simulink model "PMSM_Plant_Model"  (R2020a)
settings: configuration reference "SLRT" (kept outside this file)
undefined symbols (not defined in the file): adcTransducerVoltAtZeroAmpere, adcTransducerVoltPerAmpere, discInertia, encoderCountPerRevolution, encoderPositionValidAtStartup, encoderRotorPositionAtIndex, inverterBusVoltage, pmsmCoulombFrictionTorque, pmsmInductanceL0, pmsmInertia, pmsmPolePairs, pmsmRotorPositionInit, pmsmTorqueConstant, pmsmViscousFrictionCoefficient, pwmCounterMax, sampleTimeCurrentControl
libraries: fl_lib x15, nesl_utility x14, ee_lib x6, autolibpmsmexterior x2, utils_lib x1, mcbplantlib x1, autolibinverter x1, RotationalFrictionBrake_lib x1, eeTransforms x1
settings Model: DataDictionary=pmsmPlantData.sldd  EnableAccessToBaseWorkspace=off  DataTypeOverride=Off  VariantConfigurationObject=pmsmPlantVarObj  OrderedModelArguments=off  Creator=promero  LastModifiedBy=manuel.fedou
settings ConfigSetRef: SourceName=SLRT

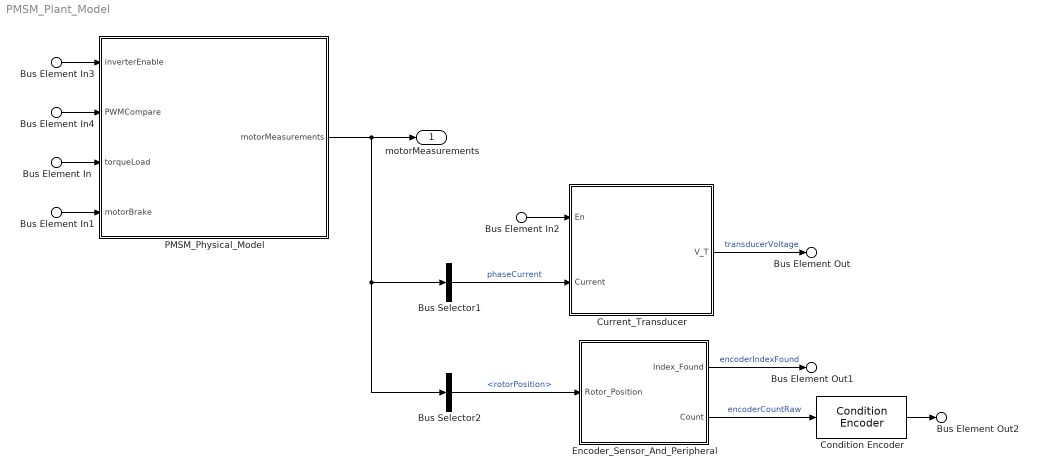
== system PMSM_Plant_Model ==
  Bus Element In : Inport  PortName=inputs  Element=torqueLoad
  Bus Element In2 : Inport  PortName=inputs  Element=connectCurrentSensor
  Bus Element In1 : Inport  PortName=inputs  Element=motorBrake
  Bus Element In3 : Inport  Port=2  PortName=commands  Element=inverterEnable
  Bus Element In4 : Inport  Port=2  PortName=commands  Element=pwmCompare
  Bus Selector1 : BusSelector  OutputSignals=phaseCurrentA,phaseCurrentB  OutputAsBus=on
  Bus Selector2 : BusSelector  OutputSignals=rotorPosition
  Condition Encoder : utils_lib/Condition Encoder  cntsPerRevolution=encoderCountPerRevolution  positiveDirection=encoderALeadsB
  Current_Transducer : Subsystem
      mask Display: image('currentTransducerMask.png');
  Encoder_Sensor_And_Peripheral : Subsystem
      mask Display:
      | image('encoderSensorAndPeripheralMask.png')
      | port_label('input',1,'P')
      | port_label('output',1,sprintf('Index\nFound'))
      | port_label('output',2,'Count')
  PMSM_Physical_Model : Subsystem  Variant=on  VariantControl=Choice
      mask Display: image('focVelocityMotorAndLoadMask.png'); % Use "Edit Image" on toolstrip to change.
  motorMeasurements : Outport  OutDataTypeStr=Bus: motorMeasurements  VectorParamsAs1DForOutWhenUnconnected=off
  Bus Element Out : Outport  Port=2  PortName=feedback  Element=transducerVoltage
  Bus Element Out1 : Outport  Port=2  PortName=feedback  Element=encoderIndexFound
  Bus Element Out2 : Outport  Port=2  PortName=feedback  Element=encoderCount
  wires:
  Bus Selector2/1 -> Encoder_Sensor_And_Peripheral/1(Rotor_Position)  "<rotorPosition>"
  Encoder_Sensor_And_Peripheral/2(Count) -> Condition Encoder/1  "encoderCountRaw"
  PMSM_Physical_Model/1(motorMeasurements) -> motorMeasurements/1, Bus Selector2/1, Bus Selector1/1
  Bus Element In3/1 -> PMSM_Physical_Model/1(inverterEnable)
  Bus Element In4/1 -> PMSM_Physical_Model/2(PWMCompare)
  Bus Selector1/1 -> Current_Transducer/2(Current)  "phaseCurrent"
  Bus Element In/1 -> PMSM_Physical_Model/3(torqueLoad)
  Bus Element In1/1 -> PMSM_Physical_Model/4(motorBrake)
  Bus Element In2/1 -> Current_Transducer/1(En)
  Current_Transducer/1(V_T) -> Bus Element Out/1  "transducerVoltage"
  Encoder_Sensor_And_Peripheral/1(Index_Found) -> Bus Element Out1/1  "encoderIndexFound"
  Condition Encoder/1 -> Bus Element Out2/1

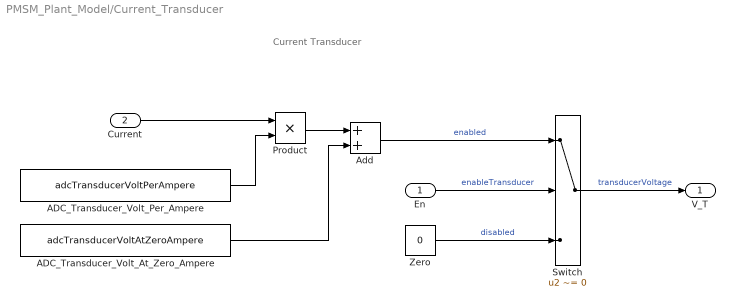
== system PMSM_Plant_Model/Current_Transducer ==
  note: Current Transducer
  En : Inport
  Current : Inport  Port=2
  ADC_Transducer_Volt_At_Zero_Ampere : Constant  Value=adcTransducerVoltAtZeroAmpere
  ADC_Transducer_Volt_Per_Ampere : Constant  Value=adcTransducerVoltPerAmpere
  Add : Sum
  Product : Product  RndMeth=Zero
  Switch : Switch  Criteria=u2 ~= 0  OutDataTypeStr=Inherit: Inherit via back propagation
  Zero : Constant  Value=0
  V_T : Outport  VectorParamsAs1DForOutWhenUnconnected=off
  wires:
  Current/1 -> Product/1
  ADC_Transducer_Volt_At_Zero_Ampere/1 -> Add/2
  Product/1 -> Add/1
  ADC_Transducer_Volt_Per_Ampere/1 -> Product/2
  Zero/1 -> Switch/3  "disabled"
  Switch/1 -> V_T/1  "transducerVoltage"
  Add/1 -> Switch/1  "enabled"
  En/1 -> Switch/2  "enableTransducer"

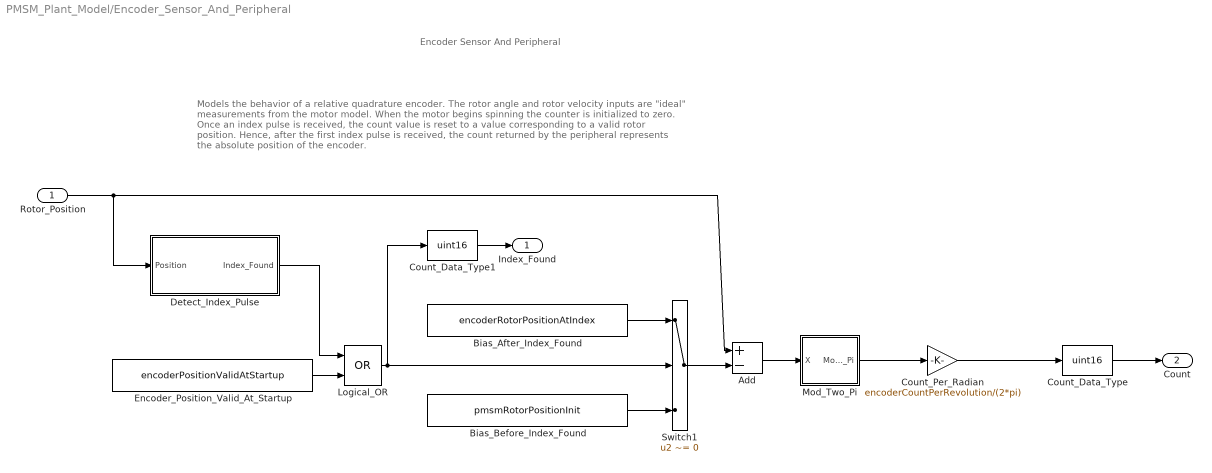
== system PMSM_Plant_Model/Encoder_Sensor_And_Peripheral ==
  note: Models the behavior of a relative quadrature encoder. The rotor angle and rotor velocity inputs are "ideal" measurements from the motor model.
      | When the motor begins spinning the counter is initialized to zero.
      | Once an index pulse is received, the count value is reset to a value corresponding to a valid rotor position.
      | Hence, after the first index pulse is received, the count returned by the peripheral represents the absolute position of the encoder.
  note: Encoder Sensor And Peripheral
  Rotor_Position : Inport
  Add : Sum  Inputs=+-
  Bias_After_Index_Found : Constant  Value=encoderRotorPositionAtIndex
  Bias_Before_Index_Found : Constant  Value=pmsmRotorPositionInit
  Count_Data_Type : DataTypeConversion  OutDataTypeStr=uint16
  Count_Data_Type1 : DataTypeConversion  OutDataTypeStr=uint16
  Count_Per_Radian : Gain  Gain=encoderCountPerRevolution/(2*pi)
      settings: AttributesFormatString=|
      | ------------------------------------------
      | Gain = %<Gain>
  Detect_Index_Pulse : Subsystem
  Encoder_Position_Valid_At_Startup : Constant  Value=encoderPositionValidAtStartup
  Logical_OR : Logic  Operator=OR  IconShape=distinctive  AllPortsSameDT=off  OutDataTypeStr=boolean
  Mod_Two_Pi : Subsystem
      mask Display:
      | text(0.5, 0.5,'Mod 2\pi',...
      |   'HorizontalAlignment', 'Center',...
      |   'VerticalAlignment', 'Middle',...
      |   'texmode', 'on')
  Switch1 : Switch  Criteria=u2 ~= 0
  Index_Found : Outport  VectorParamsAs1DForOutWhenUnconnected=off
  Count : Outport  Port=2  VectorParamsAs1DForOutWhenUnconnected=off
  wires:
  Bias_Before_Index_Found/1 -> Switch1/3
  Bias_After_Index_Found/1 -> Switch1/1
  Logical_OR/1 -> Count_Data_Type1/1, Switch1/2
  Encoder_Position_Valid_At_Startup/1 -> Logical_OR/2
  Detect_Index_Pulse/1(Index_Found) -> Logical_OR/1
  Rotor_Position/1 -> Add/1, Detect_Index_Pulse/1(Position)
  Mod_Two_Pi/1(Mod_X_Two_Pi) -> Count_Per_Radian/1
  Count_Data_Type/1 -> Count/1
  Switch1/1 -> Add/2
  Add/1 -> Mod_Two_Pi/1(X)
  Count_Per_Radian/1 -> Count_Data_Type/1
  Count_Data_Type1/1 -> Index_Found/1

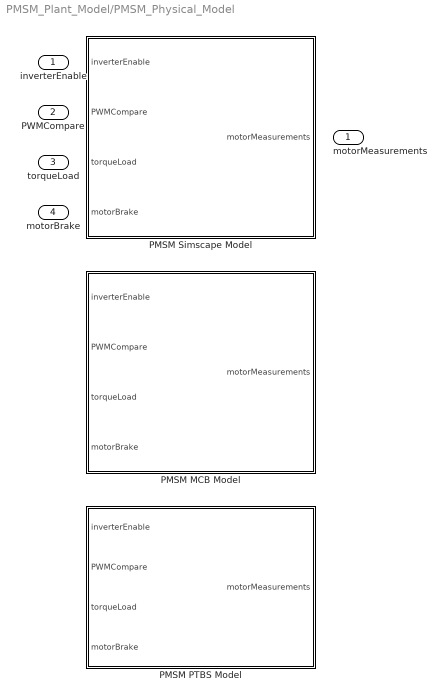
== system PMSM_Plant_Model/PMSM_Physical_Model ==
  inverterEnable : Inport
  PWMCompare : Inport  Port=2
  torqueLoad : Inport  Port=3
  motorBrake : Inport  Port=4
  PMSM MCB Model : Subsystem  VariantControl=MCBPlant
  PMSM PTBS Model : Subsystem  VariantControl=PTBSPlant
  PMSM Simscape Model : Subsystem  VariantControl=SimscapePlant
  motorMeasurements : Outport

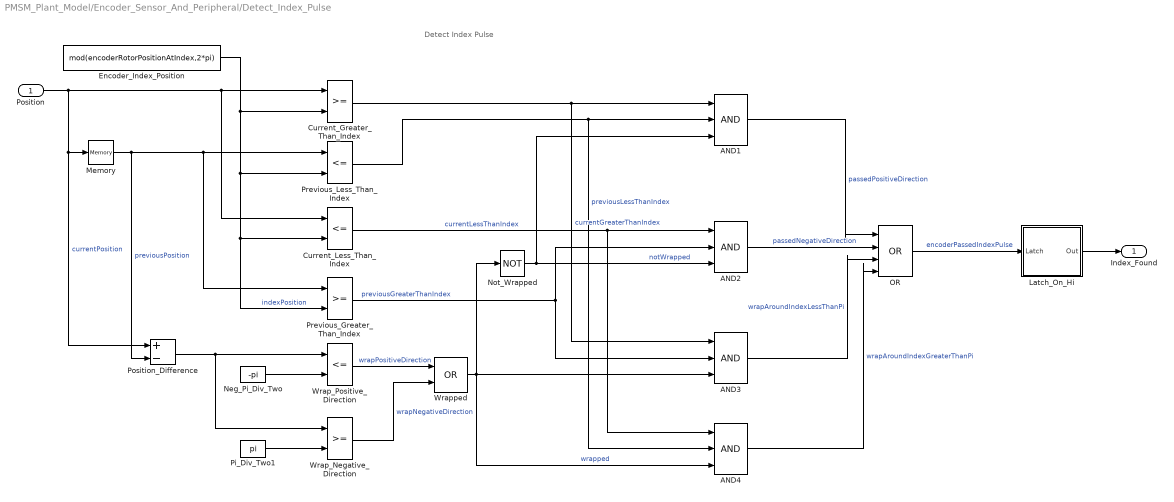
== system PMSM_Plant_Model/Encoder_Sensor_And_Peripheral/Detect_Index_Pulse ==
  note: Detect Index Pulse
  Position : Inport
  AND{1..4} (4 alike) : Logic  Inputs=3  IconShape=distinctive  AllPortsSameDT=off  OutDataTypeStr=boolean
  Current_Greater_Than_Index : RelationalOperator  OutDataTypeStr=boolean  RndMeth=Nearest
  Current_Less_Than_Index : RelationalOperator  Operator=<=  OutDataTypeStr=boolean  RndMeth=Nearest
  Encoder_Index_Position : Constant  Value=mod(encoderRotorPositionAtIndex,2*pi)
  Latch_On_Hi : Subsystem
  Memory : Memory  InitialCondition=pmsmRotorPositionInit  LinearizeAsDelay=on
  Neg_Pi_Div_Two : Constant  Value=-pi
  Not_Wrapped : Logic  Operator=NOT  IconShape=distinctive  AllPortsSameDT=off  OutDataTypeStr=boolean
  OR : Logic  Operator=OR  Inputs=4  IconShape=distinctive  AllPortsSameDT=off  OutDataTypeStr=boolean
  Pi_Div_Two1 : Constant  Value=pi
  Position_Difference : Sum  Inputs=+-
  Previous_Greater_Than_Index : RelationalOperator  OutDataTypeStr=boolean  RndMeth=Nearest
  Previous_Less_Than_Index : RelationalOperator  Operator=<=  OutDataTypeStr=boolean  RndMeth=Nearest
  Wrap_Negative_Direction : RelationalOperator  OutDataTypeStr=boolean  RndMeth=Nearest
  Wrap_Positive_Direction : RelationalOperator  Operator=<=  OutDataTypeStr=boolean  RndMeth=Nearest
  Wrapped : Logic  Operator=OR  IconShape=distinctive  AllPortsSameDT=off  OutDataTypeStr=boolean
  Index_Found : Outport  VectorParamsAs1DForOutWhenUnconnected=off
  wires:
  AND2/1 -> OR/2  "passedNegativeDirection"
  AND1/1 -> OR/1  "passedPositiveDirection"
  Current_Less_Than_Index/1 -> AND2/1, AND4/1  "currentLessThanIndex"
  Previous_Greater_Than_Index/1 -> AND2/2, AND3/2  "previousGreaterThanIndex"
  OR/1 -> Latch_On_Hi/1(Latch)  "encoderPassedIndexPulse"
  Encoder_Index_Position/1 -> Previous_Less_Than_Index/2, Previous_Greater_Than_Index/2, Current_Less_Than_Index/2, Current_Greater_Than_Index/2  "indexPosition"
  Previous_Less_Than_Index/1 -> AND1/2, AND4/2  "previousLessThanIndex"
  Current_Greater_Than_Index/1 -> AND3/1, AND1/1  "currentGreaterThanIndex"
  Memory/1 -> Position_Difference/2, Previous_Greater_Than_Index/1, Previous_Less_Than_Index/1  "previousPosition"
  Position/1 -> Memory/1, Position_Difference/1, Current_Less_Than_Index/1, Current_Greater_Than_Index/1  "currentPosition"
  Position_Difference/1 -> Wrap_Negative_Direction/1, Wrap_Positive_Direction/1
  Wrap_Positive_Direction/1 -> Wrapped/1  "wrapPositiveDirection"
  Neg_Pi_Div_Two/1 -> Wrap_Positive_Direction/2
  Wrap_Negative_Direction/1 -> Wrapped/2  "wrapNegativeDirection"
  Pi_Div_Two1/1 -> Wrap_Negative_Direction/2
  AND3/1 -> OR/3  "wrapAroundIndexLessThanPi"
  Latch_On_Hi/1(Out) -> Index_Found/1
  Not_Wrapped/1 -> AND1/3, AND2/3  "notWrapped"
  Wrapped/1 -> AND4/3, AND3/3, Not_Wrapped/1  "wrapped"
  AND4/1 -> OR/4  "wrapAroundIndexGreaterThanPi"

== system PMSM_Plant_Model/Encoder_Sensor_And_Peripheral/Mod_Two_Pi ==
  note: Mod Two Pi
  X : Inport
  Mod : Math  Operator=mod  SignedPower=on  SaturateOnIntegerOverflow=on
  Two_Pi : Constant  Value=2*pi  OutDataTypeStr=Inherit: Inherit via back propagation
  Mod_X_Two_Pi : Outport  VectorParamsAs1DForOutWhenUnconnected=off
  wires:
  X/1 -> Mod/1
  Two_Pi/1 -> Mod/2
  Mod/1 -> Mod_X_Two_Pi/1

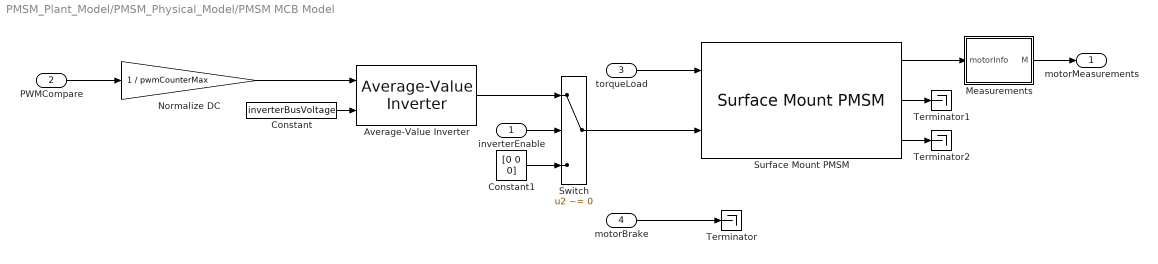
== system PMSM_Plant_Model/PMSM_Physical_Model/PMSM MCB Model ==
  inverterEnable : Inport
  PWMCompare : Inport  Port=2
  torqueLoad : Inport  Port=3
  motorBrake : Inport  Port=4
  Average-Value Inverter : mcbplantlib/Average-Value Inverter
  Constant : Constant  Value=inverterBusVoltage
  Constant1 : Constant  Value=[0 0 0]
  Measurements : Subsystem
  Normalize DC : Gain  Gain=1 / pwmCounterMax  OutDataTypeStr=double
  Surface Mount PMSM : autolibpmsmexterior/Surface Mount PMSM  port_config=Torque  sim_type=Discrete  Ts=sampleTimeCurrentControl  P=pmsmPolePairs  Rs=pmsmStatorPhaseResistance  Ldq_=pmsmInductanceLd  KConstText=Torque constant (Kt):  lambda_pm=pmsmFluxLinkage  Ke=159.9771  Kt=pmsmTorqueConstant  mechanical=[pmsmInertia+discInertia, pmsmViscousFrictionCoefficient, pmsmCoulombFrictionTorque]  idq0=[pmsmInductanceL0 pmsmInductanceL0]  theta_init=pmsmRotorPositionInit - 2*pi  omega_init=pmsmRotorVelocityInit  KConst=pmsmTorqueConstant  lambda_pm_calc=0.005  RefBlkName='autolibpmsmexterior/Surface Mount PMSM'  aMode=5  Ldq="[0.0017      0.0017]"
      settings: SourceProductBaseCode=PW,MT,UV,VE,VP
  Switch : Switch  Criteria=u2 ~= 0
  Terminator : Terminator
  Terminator1 : Terminator
  Terminator2 : Terminator
  motorMeasurements : Outport  VectorParamsAs1DForOutWhenUnconnected=off
  wires:
  motorBrake/1 -> Terminator/1
  Surface Mount PMSM/1 -> Measurements/1(motorInfo)
  Measurements/1(M) -> motorMeasurements/1
  inverterEnable/1 -> Switch/2
  Constant1/1 -> Switch/3
  torqueLoad/1 -> Surface Mount PMSM/1
  Constant/1 -> Average-Value Inverter/2
  Switch/1 -> Surface Mount PMSM/2
  Average-Value Inverter/1 -> Switch/1
  Surface Mount PMSM/2 -> Terminator1/1
  Surface Mount PMSM/3 -> Terminator2/1
  Normalize DC/1 -> Average-Value Inverter/1
  PWMCompare/1 -> Normalize DC/1

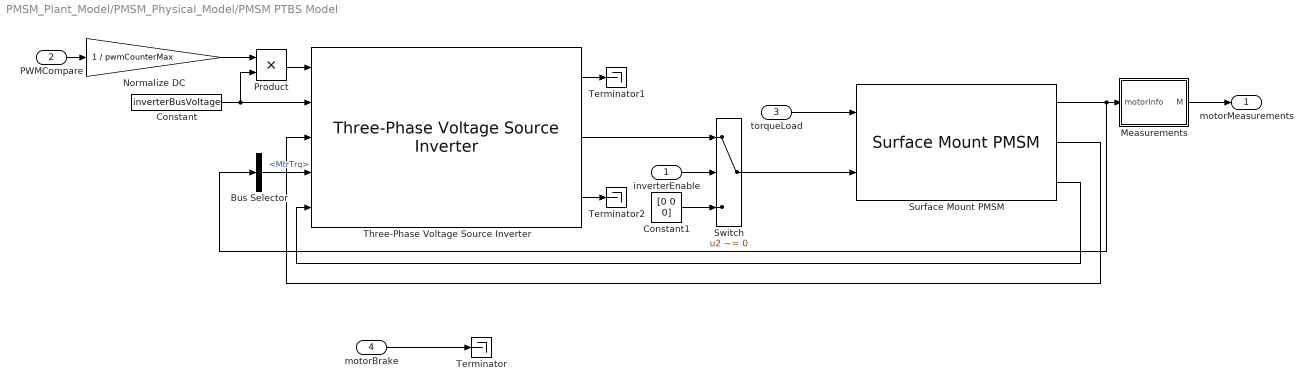
== system PMSM_Plant_Model/PMSM_Physical_Model/PMSM PTBS Model ==
  inverterEnable : Inport
  PWMCompare : Inport  Port=2
  torqueLoad : Inport  Port=3
  motorBrake : Inport  Port=4
  Bus Selector : BusSelector  OutputSignals=MtrTrq
  Constant : Constant  Value=inverterBusVoltage
  Constant1 : Constant  Value=[0 0 0]
  Measurements : Subsystem
  Normalize DC : Gain  Gain=1 / pwmCounterMax  OutDataTypeStr=double
  Product : Product
  Surface Mount PMSM : autolibpmsmexterior/Surface Mount PMSM  port_config=Torque  sim_type=Discrete  Ts=sampleTimeCurrentControl  P=pmsmPolePairs  Rs=pmsmStatorPhaseResistance  Ldq_=pmsmInductanceLd  KConstText=Torque constant (Kt):  lambda_pm=pmsmFluxLinkage  Ke=159.9771  Kt=pmsmTorqueConstant  mechanical=[pmsmInertia+discInertia, pmsmViscousFrictionCoefficient, pmsmCoulombFrictionTorque]  idq0=[pmsmInductanceL0 pmsmInductanceL0]  theta_init=pmsmRotorPositionInit - 2*pi  omega_init=pmsmRotorVelocityInit  KConst=pmsmTorqueConstant  lambda_pm_calc=0.005  RefBlkName='autolibpmsmexterior/Surface Mount PMSM'  aMode=5  Ldq="[0.0017      0.0017]"
      settings: SourceProductBaseCode=PW,MT,UV,VE,VP
  Switch : Switch  Criteria=u2 ~= 0
  Terminator : Terminator
  Terminator1 : Terminator
  Terminator2 : Terminator
  Three-Phase Voltage Source Inverter : autolibinverter/Three-Phase Voltage Source Inverter  InvrtrTmpInpEnbl=off  enable_hdl=off  model_type=Commanded phase voltage  fs=10000  w_eff_bp=[-1000 -500 0 500 1000]  n1=128  T_eff_bp=[-200 -100 0 100 200]  Temp_eff_bp=[213.15 293.15 373.15]  n2=128  ploss_table=[1 0.999 0.989 0.997 0.996;0.995 0.994 0.993 0.992 0.991;0.990 0.989 0.988 0.987 0.986;0.985 0.984 0.983 0.982 0.981;0.980 0.979 0.978 0.977 0.976]  ploss_table_3d=cat(3,0.95*[1 0.999 0.989 0.997 0.996;0.995 0.994 0.993 0.992 0.991;0.990 0.989 0.988 0.987 0.986;0.985 0.984 0.983 0.982 0.981;0.980 0.979 0.978 0.977 0.976],[1 0.999 0.989 0.997 0.996;0.995 0.994 0.993 0.992 0.991;0.990 0.989 0.988 0.987 0.986;0.985 0.984 0.983 0.982 0.981;0.980 0.979 0.978 0.977 0.976],0.92*[1 0.999 0.989 0.997 0.996;0.995 0.994 0.993 0.992 0.991;0.990 0.989 0.988 0.987 0.986;0.985 0.984 0.983 0.982 0.981;0.980 0.979 0.978 0.977 0.976])  preExtrapFlag=off  u1max=1000  u1min=-1000  u2max=200  u2min=-200  intPrec=23  RefBlkName='autolibmappedmotor/Mapped Motor'  CalLossMapData={}  CalLossWithTempMapData={}
      settings: SourceProductBaseCode=PW,MT,UV,VE,VP
  motorMeasurements : Outport  VectorParamsAs1DForOutWhenUnconnected=off
  wires:
  Surface Mount PMSM/2 -> Three-Phase Voltage Source Inverter/3
  inverterEnable/1 -> Switch/2
  Constant1/1 -> Switch/3
  motorBrake/1 -> Terminator/1
  torqueLoad/1 -> Surface Mount PMSM/1
  Switch/1 -> Surface Mount PMSM/2
  PWMCompare/1 -> Normalize DC/1
  Measurements/1(M) -> motorMeasurements/1
  Three-Phase Voltage Source Inverter/2 -> Switch/1
  Surface Mount PMSM/3 -> Three-Phase Voltage Source Inverter/5
  Three-Phase Voltage Source Inverter/1 -> Terminator1/1
  Three-Phase Voltage Source Inverter/3 -> Terminator2/1
  Constant/1 -> Product/2, Three-Phase Voltage Source Inverter/2
  Surface Mount PMSM/1 -> Bus Selector/1, Measurements/1(motorInfo)
  Bus Selector/1 -> Three-Phase Voltage Source Inverter/4  "<MtrTrq>"
  Product/1 -> Three-Phase Voltage Source Inverter/1
  Normalize DC/1 -> Product/1

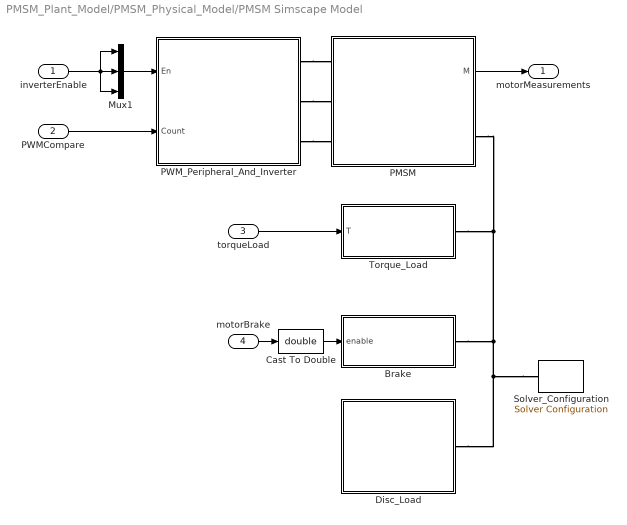
== system PMSM_Plant_Model/PMSM_Physical_Model/PMSM Simscape Model ==
  inverterEnable : Inport
  PWMCompare : Inport  Port=2
  torqueLoad : Inport  Port=3
  motorBrake : Inport  Port=4
  Brake : Subsystem
  Cast To Double : DataTypeConversion  OutDataTypeStr=double
  Disc_Load : Subsystem  VariantControl=loadType == motorLoad.disc
      mask Display: image('discAluminumMask.png')
  Mux1 : Mux  Inputs=3
  PMSM : Subsystem
      mask Display:
      | image('pmsmMask.png')
      | text(0.03, 0.80, 'A', 'HorizontalAlignment', 'Left')
      | text(0.03, 0.50, 'B', 'HorizontalAlignment', 'Left')
      | text(0.03, 0.20, 'C', 'HorizontalAlignment', 'Left')
      | text(0.98, 0.75, 'M', 'HorizontalAlignment', 'Right')
      | text(0.98, 0.25, 'R', 'HorizontalAlignment', 'Right')
  PWM_Peripheral_And_Inverter : Subsystem  VariantControl=variantPwm == enumPwm.behavior
      mask Display: image('pwmPeripheralAndInverterMask.png');
  Solver_Configuration : nesl_utility/Solver Configuration  PhysicalDomain=network_engine_domain  SubClassName=solver  LeftPortType=input  RightPortType=generic  Tones=[]  Harmonics=[]  SimulateNoise=off  Profile=off  UseLocalSampling=off  EnableSwitchedLinearOptims=on  FrequencyDomain=off  UseCCode=off  RelTol=0.001  AbsTol=1e-06  MinStep=1e-09  ToWorkspace=off  RevertToSquareIcSolve=off  NumHomotopyIterations=100  PhasorMode=off  PhasorModeNumHarmonics=1  DoDC=off  ResidualTolerance=1e-9  UseLocalSolver=on  LocalSolverChoice=NE_TRAPEZOIDAL_ADVANCER  LocalSolverSampleTime=sampleTimeCurrentControl  DoFixedCost=on  MaxNonlinIter=1  MaxModeIter=2  LinearAlgebra=auto  EquationFormulation=NE_TIME_EF  DelaysMemoryBudget=1024  AutomaticFiltering=on  FilteringTimeConstant=0.001  PartitionStorageMethod=AS_NEEDED  PartitionMemoryBudget=1024  PartitionMethod=FAST
  Torque_Load : Subsystem  VariantControl=loadType == motorLoad.disc
      mask Display:
      | image('torqueLoadMask.png')
      | text(0.03, 0.5, 'T', 'HorizontalAlignment', 'Left')
      | text(0.98, 0.5, 'R', 'HorizontalAlignment', 'Right')
  motorMeasurements : Outport  VectorParamsAs1DForOutWhenUnconnected=off
  wires:
  PWMCompare/1 -> PWM_Peripheral_And_Inverter/2(Count)
  torqueLoad/1 -> Torque_Load/1(T)
  PMSM/1(M) -> motorMeasurements/1
  motorBrake/1 -> Cast To Double/1
  Mux1/1 -> PWM_Peripheral_And_Inverter/1(En)
  inverterEnable/1 -> Mux1/3, Mux1/1, Mux1/2
  Cast To Double/1 -> Brake/1(enable)
  connections:
  Solver_Configuration/RConn1 -- PMSM/RConn1 -- Torque_Load/RConn1 -- Brake/RConn1 -- Disc_Load/RConn1
  PWM_Peripheral_And_Inverter/RConn3 -- PMSM/LConn3
  PWM_Peripheral_And_Inverter/RConn2 -- PMSM/LConn2
  PWM_Peripheral_And_Inverter/RConn1 -- PMSM/LConn1

== system PMSM_Plant_Model/Encoder_Sensor_And_Peripheral/Detect_Index_Pulse/Latch_On_Hi ==
  note: Latch On Hi
  Latch : Inport
  Memory : Memory  LinearizeAsDelay=on
  One : Constant  OutDataTypeStr=boolean
  Switch : Switch  Criteria=u2 ~= 0  Threshold=1
  Out : Outport  VectorParamsAs1DForOutWhenUnconnected=off
  wires:
  Switch/1 -> Out/1, Memory/1
  Latch/1 -> Switch/3
  One/1 -> Switch/1
  Memory/1 -> Switch/2

== system PMSM_Plant_Model/PMSM_Physical_Model/PMSM MCB Model/Measurements ==
  note: Measurements
  motorInfo : Inport
  Bus Selector : BusSelector  OutputSignals=IaStator,IbStator,IcStator,IdSync,IqSync,MtrTrq,MtrPos,MtrSpd
  Bus_Creator2 : BusCreator  Inputs=10  OutDataTypeStr=Bus: motorMeasurements
      settings: InheritFromInputs=off
  Gain1 : Gain  Gain=pmsmPolePairs
      settings: AttributesFormatString=-----------------------------\n%<Gain>
  Gain2 : Gain  Gain=pmsmPolePairs
      settings: AttributesFormatString=-----------------------------\n%<Gain>
  M : Outport  OutDataTypeStr=Bus: motorMeasurements  VectorParamsAs1DForOutWhenUnconnected=off
  wires:
  Bus_Creator2/1 -> M/1
  Bus Selector/1 -> Bus_Creator2/1  "<IaStator>"
  Bus Selector/3 -> Bus_Creator2/3  "<IcStator>"
  Bus Selector/2 -> Bus_Creator2/2  "<IbStator>"
  motorInfo/1 -> Bus Selector/1
  Bus Selector/4 -> Bus_Creator2/4  "<IdSync>"
  Bus Selector/5 -> Bus_Creator2/5  "<IqSync>"
  Bus Selector/6 -> Bus_Creator2/6  "<MtrTrq>"
  Bus Selector/7 -> Gain1/1, Bus_Creator2/7  "<MtrPos>"
  Gain1/1 -> Bus_Creator2/8
  Bus Selector/8 -> Gain2/1, Bus_Creator2/9  "<MtrSpd>"
  Gain2/1 -> Bus_Creator2/10  "electricalVelocity"

== system PMSM_Plant_Model/PMSM_Physical_Model/PMSM PTBS Model/Measurements ==
  note: Measurements
  motorInfo : Inport
  Bus Selector : BusSelector  OutputSignals=IaStator,IbStator,IcStator,IdSync,IqSync,MtrTrq,MtrPos,MtrSpd
  Bus_Creator2 : BusCreator  Inputs=10  OutDataTypeStr=Bus: motorMeasurements
      settings: InheritFromInputs=off
  Gain1 : Gain  Gain=pmsmPolePairs
      settings: AttributesFormatString=-----------------------------\n%<Gain>
  Gain2 : Gain  Gain=pmsmPolePairs
      settings: AttributesFormatString=-----------------------------\n%<Gain>
  M : Outport  OutDataTypeStr=Bus: motorMeasurements  VectorParamsAs1DForOutWhenUnconnected=off
  wires:
  Bus_Creator2/1 -> M/1
  Bus Selector/1 -> Bus_Creator2/1  "<IaStator>"
  Bus Selector/3 -> Bus_Creator2/3  "<IcStator>"
  Bus Selector/2 -> Bus_Creator2/2  "<IbStator>"
  motorInfo/1 -> Bus Selector/1
  Bus Selector/4 -> Bus_Creator2/4  "<IdSync>"
  Bus Selector/5 -> Bus_Creator2/5  "<IqSync>"
  Bus Selector/6 -> Bus_Creator2/6  "<MtrTrq>"
  Bus Selector/7 -> Gain1/1, Bus_Creator2/7  "<MtrPos>"
  Gain1/1 -> Bus_Creator2/8
  Bus Selector/8 -> Gain2/1, Bus_Creator2/9  "<MtrSpd>"
  Gain2/1 -> Bus_Creator2/10  "electricalVelocity"

== system PMSM_Plant_Model/PMSM_Physical_Model/PMSM Simscape Model/Brake ==
  enable : Inport
  Mechanical Rotational Reference2 : fl_lib/Mechanical/Rotational Elements/Mechanical Rotational Reference
  Rotational Friction Brake : RotationalFrictionBrake_lib/Rotational Friction Brake  brkwy_trq=25 N*m  Col_trq=20 N*m  visc_coef=0.001 N*m/(rad/s)  trans_coef=10 s/rad  vel_thr=1e-4 rad/s  w_specify=off  w_priority=None  w=0 rad/s  w_nominal_specify=off  w_nominal_unit=rad/s  w_nominal_value=1  t_specify=off  t_priority=None  t=0 N*m  t_nominal_specify=off  t_nominal_unit=N*m  t_nominal_value=1
      settings: InternalSimscapePortConfiguration="{\"Bottom\":[],\"Left\":[{\"id\":\"R\",\"label\":\"R\",\"type\":\"foundation.mechanical.rotational.rotational\"}],\"Right\":[{\"id\":\"C\",\"label\":\"C\",\"type\":\"foundation.mechanical.rotational.rotational\"},{\"id\":\"S\",\"label\":\"S\",\"type\":\"input\"}],\"Top\":[]}"
  Simulink-PS Converter : nesl_utility/Simulink-PS Converter  PhysicalDomain=network_engine_domain  SubClassName=ps_input  LeftPortType=input  RightPortType=output  PseudoPeriodic=off  Frequencies=[]  NoiseDistribution=none  NoiseParameters=[]  Unit=1  AffineConversion=off  FilteringAndDerivatives=zero  SimscapeFilterOrder=1  InputFilterTimeConstant=0.001  UdotUserProvided=0
  Brake Torque : PMIOPort  Side=Right
  wires:
  enable/1 -> Simulink-PS Converter/1
  connections:
  Simulink-PS Converter/RConn1 -- Rotational Friction Brake/RConn2
  Rotational Friction Brake/LConn1 -- Brake Torque/RConn1
  Mechanical Rotational Reference2/LConn1 -- Rotational Friction Brake/RConn1

== system PMSM_Plant_Model/PMSM_Physical_Model/PMSM Simscape Model/Disc_Load ==
  note: Disc Load
  Inertia : fl_lib/Mechanical/Rotational Elements/Inertia  inertia=discInertia kg*m^2  w_specify=off  w_priority=None  w=pmsm.RotorVelocityInit rad/s  w_nominal_specify=off  w_nominal_unit=rad/s  w_nominal_value=1  t_specify=off  t_priority=High  t=0 N*m  t_nominal_specify=off  t_nominal_unit=N*m  t_nominal_value=1
      settings: AttributesFormatString=|
      | ---------------------------
      | Inertia = %<inertia>
  R : PMIOPort  Side=Right
  connections:
  Inertia/LConn1 -- R/RConn1

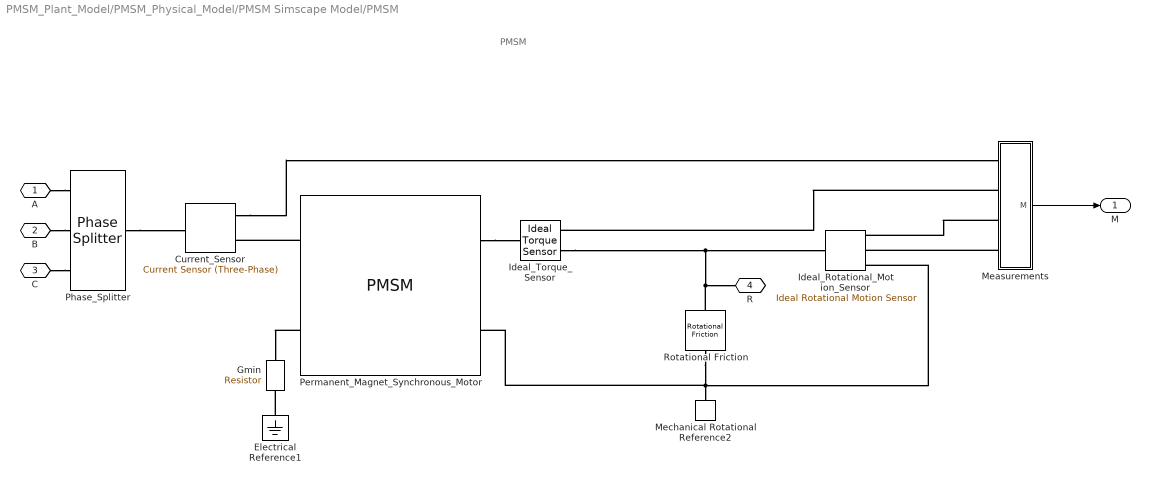
== system PMSM_Plant_Model/PMSM_Physical_Model/PMSM Simscape Model/PMSM ==
  note: PMSM
  Current_Sensor : ee_lib/Sensors & Transducers/Current Sensor (Three-Phase)
  Electrical Reference1 : fl_lib/Electrical/Electrical Elements/Electrical Reference
  Gmin : fl_lib/Electrical/Electrical Elements/Resistor  R=1e9 Ohm  i_specify=off  i_priority=None  i=0 A  i_nominal_specify=off  i_nominal_unit=A  i_nominal_value=1  v_specify=off  v_priority=None  v=0 V  v_nominal_specify=off  v_nominal_unit=V  v_nominal_value=1
  Ideal_Rotational_Mot ion_Sensor : fl_lib/Mechanical/Mechanical Sensors/Ideal Rotational Motion Sensor  wrap_angle=simscape.enum.onoff.on  offset=pmsmRotorPositionInit rad
  Ideal_Torque_Sensor : fl_lib/Mechanical/Mechanical Sensors/Ideal Torque Sensor
  Measurements : Subsystem
  Mechanical Rotational Reference2 : fl_lib/Mechanical/Rotational Elements/Mechanical Rotational Reference
  Permanent_Magnet_Synchronous_Motor : ee_lib/Electromechanical/Permanent Magnet/PMSM  winding_type=ee.enum.statorconnection.wye  machine_param=ee.enum.pmsm.parameterization.constant  nPolePairs=pmsmPolePairs  pmflux_param=ee.enum.pmflux.torqueconstant  pm_flux_linkage=pmsmFluxLinkage Wb  torque_constant=pmsmTorqueConstant N*m/A  back_emf_constant=0.18 V/(rad/s)  stator_param=ee.enum.statorparam.LdLqL0  Ld=pmsmInductanceLd H  Lq=pmsmInductanceLq H  idVec=[-200, 0, 200] A  iqVec=[-200, 0, 200] A  LdMatrix=0.0002 * ones(3, 3) H  LqMatrix=0.0002 * ones(3, 3) H  PmMatrix=0.1 * ones(3, 3) Wb  ktMatrix=0.18 * ones(3, 3) N*m/A  keMatrix=0.18 * ones(3, 3) V/(rad/s)  L0=pmsmInductanceL0 H  Ls=0.0002 H  Lm=0 H  Ms=0 H  Rs=pmsmStatorPhaseResistance Ohm  zero_sequence=ee.enum.park.zerosequence.include  J=pmsmInertia kg*m^2  lam=0 N*m/(rad/s)  axes_param=ee.enum.rotorangle.daxis  i_d_specify=off  i_d_priority=None  i_d=0 A  i_d_nominal_specify=off  i_d_nominal_unit=A  i_d_nominal_value=1  i_q_specify=off  i_q_priority=None  i_q=0 A  i_q_nominal_specify=off  i_q_nominal_unit=A  i_q_nominal_value=1  torque_specify=off  torque_priority=None  torque=0 N*m  torque_nominal_specify=off  torque_nominal_unit=N*m  torque_nominal_value=1  angular_velocity_specify=on  angular_velocity_priority=High  angular_velocity=pmsmRotorVelocityInit rad/s  angular_velocity_nominal_specify=off  angular_velocity_nominal_unit=rpm  angular_velocity_nominal_value=1  angular_position_specify=on  angular_position_priority=High  angular_position=pmsmRotorPositionInit rad  angular_position_nominal_specify=off  angular_position_nominal_unit=deg  angular_position_nominal_value=1  loss_param=ee.enum.ironloss.none  losses_oc=[0, 0, 0] W  losses_sc=[0, 0, 0] W  f_losses=60 Hz  Isc_losses=95 A  Tmeas=298.15 K  alpha=3.93e-3 1/K  alpha_flux=-0.001 1/K  stator_thermal_mass=100 J/K  rotor_thermal_mass=200 J/K  Rm_percent_rotor=90  Rd_percent_rotor=30  temperatureA_specify=off  temperatureA_priority=High  temperatureA=25 degC  temperatureA_nominal_specify=off  temperatureA_nominal_unit=degC  temperatureA_nominal_value=1  temperatureB_specify=off  temperatureB_priority=High  temperatureB=25 degC  temperatureB_nominal_specify=off  temperatureB_nominal_unit=degC  temperatureB_nominal_value=1  temperatureC_specify=off  temperatureC_priority=High  temperatureC=25 degC  temperatureC_nominal_specify=off  temperatureC_nominal_unit=degC  temperatureC_nominal_value=1  temperatureR_specify=off  temperatureR_priority=High  temperatureR=25 degC  temperatureR_nominal_specify=off  temperatureR_nominal_unit=degC  temperatureR_nominal_value=1
      settings: InternalSimscapePortConfiguration="{\"Bottom\":[],\"Left\":[{\"id\":\"N\",\"label\":\"~\",\"type\":\"foundation.electrical.three_phase\"},{\"id\":\"n\",\"label\":\"n\",\"type\":\"foundation.electrical.electrical\"}],\"Right\":[{\"id\":\"R\",\"label\":\"R\",\"type\":\"foundation.mechanical.rotational.rotational\"},{\"id\":\"C\",\"label\":\"C\",\"type\":\"foundation.mechanical.rotational.rotational\"}],\"Top\":[]}"
  Phase_Splitter : ee_lib/Connectors & References/Phase Splitter
      settings: SourceProductBaseCode=PS
  Rotational Friction : fl_lib/Mechanical/Rotational Elements/Rotational Friction  brkwy_trq=pmsmBreakawayFrictionTorque N*m  brkwy_vel=pmsmBreakawayFrictionVelocity rad/s  Col_trq=pmsmCoulombFrictionTorque N*m  visc_coef=pmsmViscousFrictionCoefficient N*m/(rad/s)  w_specify=off  w_priority=None  w=0 rad/s  w_nominal_specify=off  w_nominal_unit=rad/s  w_nominal_value=1  t_specify=off  t_priority=None  t=0 N*m  t_nominal_specify=off  t_nominal_unit=N*m  t_nominal_value=1
  A : PMIOPort  Side=Left
  B : PMIOPort  Port=2  Side=Left
  C : PMIOPort  Port=3  Side=Left
  R : PMIOPort  Port=4  Side=Right
  M : Outport  VectorParamsAs1DForOutWhenUnconnected=off
  wires:
  Measurements/1(M) -> M/1
  connections:
  Measurements/LConn4 -- Ideal_Rotational_Mot ion_Sensor/RConn2
  Measurements/LConn3 -- Ideal_Rotational_Mot ion_Sensor/RConn3
  Measurements/LConn2 -- Ideal_Torque_Sensor/RConn2
  Permanent_Magnet_Synchronous_Motor/LConn1 -- Current_Sensor/RConn2
  C/RConn1 -- Phase_Splitter/RConn3
  B/RConn1 -- Phase_Splitter/RConn2
  A/RConn1 -- Phase_Splitter/RConn1
  Permanent_Magnet_Synchronous_Motor/LConn2 -- Gmin/RConn1
  Permanent_Magnet_Synchronous_Motor/RConn2 -- Mechanical Rotational Reference2/LConn1 -- Rotational Friction/RConn1 -- Ideal_Rotational_Mot ion_Sensor/RConn1
  Phase_Splitter/LConn1 -- Current_Sensor/LConn1
  Current_Sensor/RConn1 -- Measurements/LConn1
  Electrical Reference1/LConn1 -- Gmin/LConn1
  Permanent_Magnet_Synchronous_Motor/RConn1 -- Ideal_Torque_Sensor/LConn1
  Ideal_Torque_Sensor/RConn1 -- Ideal_Rotational_Mot ion_Sensor/LConn1 -- Rotational Friction/LConn1 -- R/RConn1

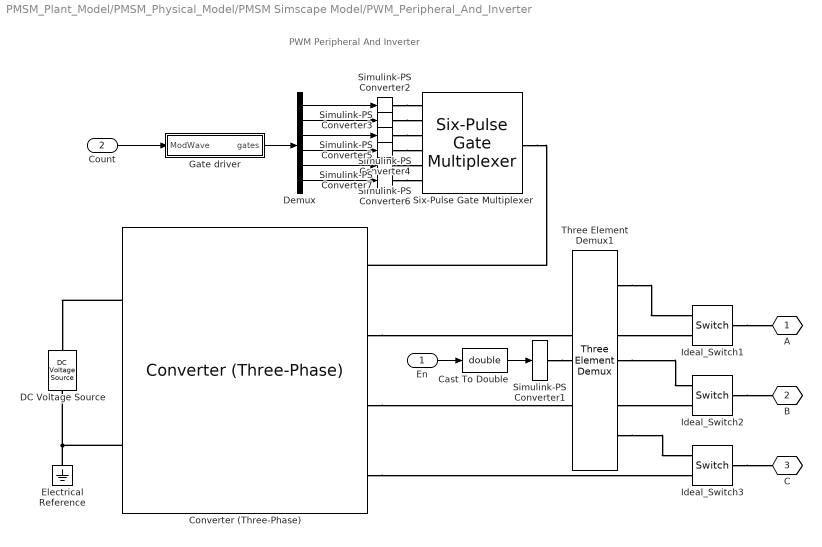
== system PMSM_Plant_Model/PMSM_Physical_Model/PMSM Simscape Model/PWM_Peripheral_And_Inverter ==
  note: PWM Peripheral And Inverter
  En : Inport
  Count : Inport  Port=2
  Cast To Double : DataTypeConversion  OutDataTypeStr=double
  Converter (Three-Phase) : ee_lib/Semiconductors & Converters/Converters/Converter (Three-Phase)  device_type=ee.enum.converters.switchingdevice.averaged  Vf=0.8 V  Ron=0.001 Ohm  Rds=0.001 Ohm  Goff=1e-6 1/Ohm  Vth=6 V  Vgt=1 V  Vgt_off=-1 V  Ih=1 A  diode_param=ee.enum.converters.protectiondiode.none  diode_Vf=0.8 V  diode_Ron=0.001 Ohm  diode_Goff=1e-5 1/Ohm  diode_C=50 nF  diode_iRM=-235 A  diode_iF=300 A  diode_idot=-50 A/us  diode_trr_param=ee.enum.converters.diodetrr.trr_factor  diode_trr_factor=3  diode_trr=15 us  diode_Qrr=1500 s*uA  snubber_type=ee.enum.converters.snubber.exclude  Rs=0.1 Ohm  Cs=1e-7 F
      settings: SourceProductBaseCode=PS  InternalSimscapePortConfiguration="{\"Bottom\":[],\"Left\":[{\"id\":\"G\",\"label\":\"G\",\"type\":\"foundation.electrical.twelve_phase\"},{\"id\":\"a\",\"label\":\"a\",\"type\":\"foundation.electrical.electrical\"},{\"id\":\"b\",\"label\":\"b\",\"type\":\"foundation.electrical.electrical\"},{\"id\":\"c\",\"label\":\"c\",\"type\":\"foundation.electrical.electrical\"}],\"Right\":[{\"id\":\"p\",\"label\":\"+\",\"type\":\"foundation.electrical.electrical\"},{\"id\":\"n\",\"label\":\"-\",\"type\":\"foundation.electrical.electrical\"}],\"Top\":[]}"
  DC Voltage Source : fl_lib/Electrical/Electrical Sources/DC Voltage Source  v0=inverterBusVoltage V
  Demux : Demux  Outputs=6
  Electrical Reference : fl_lib/Electrical/Electrical Elements/Electrical Reference
  Gate driver : Subsystem
  Ideal_Switch1 : fl_lib/Electrical/Electrical Elements/Switch  R_closed=0.0001 Ohm  G_open=1e-5 1/Ohm  Threshold=0  i_specify=off  i_priority=None  i=0 A  i_nominal_specify=off  i_nominal_unit=A  i_nominal_value=1  v_specify=off  v_priority=None  v=0 V  v_nominal_specify=off  v_nominal_unit=V  v_nominal_value=1
  Ideal_Switch2 : fl_lib/Electrical/Electrical Elements/Switch  R_closed=0.0001 Ohm  G_open=1e-5 1/Ohm  Threshold=0  i_specify=off  i_priority=None  i=0 A  i_nominal_specify=off  i_nominal_unit=A  i_nominal_value=1  v_specify=off  v_priority=None  v=0 V  v_nominal_specify=off  v_nominal_unit=V  v_nominal_value=1
  Ideal_Switch3 : fl_lib/Electrical/Electrical Elements/Switch  R_closed=0.0001 Ohm  G_open=1e-5 1/Ohm  Threshold=0  i_specify=off  i_priority=None  i=0 A  i_nominal_specify=off  i_nominal_unit=A  i_nominal_value=1  v_specify=off  v_priority=None  v=0 V  v_nominal_specify=off  v_nominal_unit=V  v_nominal_value=1
  Simulink-PS Converter1 : nesl_utility/Simulink-PS Converter  PhysicalDomain=network_engine_domain  SubClassName=ps_input  LeftPortType=input  RightPortType=output  PseudoPeriodic=off  Frequencies=[]  NoiseDistribution=none  NoiseParameters=[]  Unit=1  AffineConversion=off  FilteringAndDerivatives=zero  SimscapeFilterOrder=1  InputFilterTimeConstant=0.001  UdotUserProvided=0
  Simulink-PS Converter{2..7} (6 alike) : nesl_utility/Simulink-PS Converter  PhysicalDomain=network_engine_domain  SubClassName=ps_input  LeftPortType=input  RightPortType=output  PseudoPeriodic=off  Frequencies=[]  NoiseDistribution=none  NoiseParameters=[]  Unit=1  AffineConversion=off  FilteringAndDerivatives=provide  SimscapeFilterOrder=1  InputFilterTimeConstant=0.001  UdotUserProvided=0
  Six-Pulse Gate Multiplexer : ee_lib/Semiconductors & Converters/Converters/Six-Pulse Gate Multiplexer  R=0 Ohm
      settings: SourceProductBaseCode=PS  InternalSimscapePortConfiguration="{\"Bottom\":[],\"Left\":[{\"id\":\"GaH\",\"label\":\"Ga(H)\",\"type\":\"input\"},{\"id\":\"GaL\",\"label\":\"Ga(L)\",\"type\":\"input\"},{\"id\":\"GbH\",\"label\":\"Gb(H)\",\"type\":\"input\"},{\"id\":\"GbL\",\"label\":\"Gb(L)\",\"type\":\"input\"},{\"id\":\"GcH\",\"label\":\"Gc(H)\",\"type\":\"input\"},{\"id\":\"GcL\",\"label\":\"Gc(L)\",\"type\":\"input\"}],\"Right\":[{\"id\":\"p\",\"label\":\"G\",\"type\":\"foundation.electrical.twelve_phase\"}],\"Top\":[]}"
  Three Element Demux1 : ee_lib/Connectors & References/Three Element Demux
      settings: SourceProductBaseCode=PS  InternalSimscapePortConfiguration="{\"Bottom\":[],\"Left\":[{\"id\":\"abc\",\"label\":\"abc\",\"type\":\"input\"}],\"Right\":[{\"id\":\"a\",\"label\":\"a\",\"type\":\"output\"},{\"id\":\"b\",\"label\":\"b\",\"type\":\"output\"},{\"id\":\"c\",\"label\":\"c\",\"type\":\"output\"}],\"Top\":[]}"
  A : PMIOPort  Tag=PMCPort  Side=Right
  B : PMIOPort  Tag=PMCPort  Port=2  Side=Right
  C : PMIOPort  Tag=PMCPort  Port=3  Side=Right
  wires:
  Count/1 -> Gate driver/1(ModWave)
  En/1 -> Cast To Double/1
  Cast To Double/1 -> Simulink-PS Converter1/1
  Demux/3 -> Simulink-PS Converter4/1
  Demux/5 -> Simulink-PS Converter6/1
  Demux/4 -> Simulink-PS Converter5/1
  Demux/1 -> Simulink-PS Converter2/1
  Demux/6 -> Simulink-PS Converter7/1
  Demux/2 -> Simulink-PS Converter3/1
  Gate driver/1(gates) -> Demux/1
  connections:
  Converter (Three-Phase)/LConn3 -- Ideal_Switch2/RConn2
  Converter (Three-Phase)/LConn2 -- Ideal_Switch1/RConn2
  Simulink-PS Converter1/RConn1 -- Three Element Demux1/LConn1
  Converter (Three-Phase)/LConn4 -- Ideal_Switch3/RConn2
  Three Element Demux1/RConn3 -- Ideal_Switch3/RConn1
  Three Element Demux1/RConn2 -- Ideal_Switch2/RConn1
  Three Element Demux1/RConn1 -- Ideal_Switch1/RConn1
  Ideal_Switch3/LConn1 -- C/RConn1
  Ideal_Switch2/LConn1 -- B/RConn1
  Ideal_Switch1/LConn1 -- A/RConn1
  Converter (Three-Phase)/RConn1 -- DC Voltage Source/LConn1
  Electrical Reference/LConn1 -- Converter (Three-Phase)/RConn2 -- DC Voltage Source/RConn1
  Six-Pulse Gate Multiplexer/RConn1 -- Converter (Three-Phase)/LConn1
  Simulink-PS Converter3/RConn1 -- Six-Pulse Gate Multiplexer/LConn2
  Simulink-PS Converter5/RConn1 -- Six-Pulse Gate Multiplexer/LConn4
  Simulink-PS Converter6/RConn1 -- Six-Pulse Gate Multiplexer/LConn5
  Simulink-PS Converter7/RConn1 -- Six-Pulse Gate Multiplexer/LConn6
  Simulink-PS Converter4/RConn1 -- Six-Pulse Gate Multiplexer/LConn3
  Simulink-PS Converter2/RConn1 -- Six-Pulse Gate Multiplexer/LConn1

== system PMSM_Plant_Model/PMSM_Physical_Model/PMSM Simscape Model/Torque_Load ==
  note: Torque Load
  T : Inport
  Ideal_Torque_Source : fl_lib/Mechanical/Mechanical Sources/Ideal Torque Source
  Mechanical_Rotational_Reference : fl_lib/Mechanical/Rotational Elements/Mechanical Rotational Reference
  Simulink_PS_Converter : nesl_utility/Simulink-PS Converter  PhysicalDomain=network_engine_domain  SubClassName=ps_input  LeftPortType=input  RightPortType=output  PseudoPeriodic=off  Frequencies=[]  NoiseDistribution=none  NoiseParameters=[]  Unit=N*m  AffineConversion=off  FilteringAndDerivatives=zero  SimscapeFilterOrder=1  InputFilterTimeConstant=.001  UdotUserProvided=1
  R : PMIOPort  Side=Right
  wires:
  T/1 -> Simulink_PS_Converter/1  "loadTorque"
  connections:
  Ideal_Torque_Source/LConn1 -- R/RConn1
  Simulink_PS_Converter/RConn1 -- Ideal_Torque_Source/RConn1
  Mechanical_Rotational_Reference/LConn1 -- Ideal_Torque_Source/RConn2

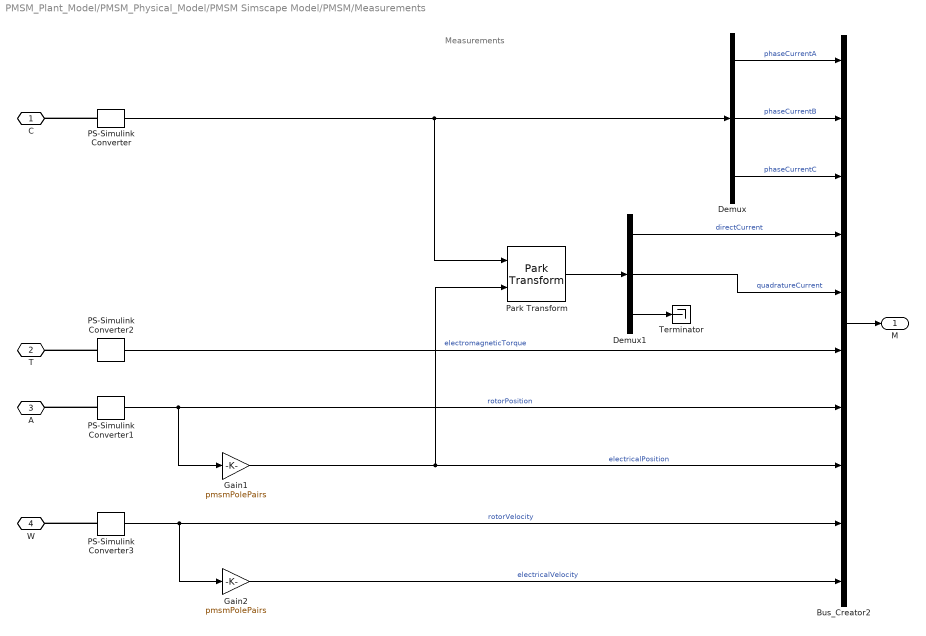
== system PMSM_Plant_Model/PMSM_Physical_Model/PMSM Simscape Model/PMSM/Measurements ==
  note: Measurements
  Bus_Creator2 : BusCreator  Inputs=10  OutDataTypeStr=Bus: motorMeasurements
      settings: InheritFromInputs=off
  Demux : Demux  Outputs=3
  Demux1 : Demux  Outputs=3
  Gain1 : Gain  Gain=pmsmPolePairs
      settings: AttributesFormatString=-----------------------------\n%<Gain>
  Gain2 : Gain  Gain=pmsmPolePairs
      settings: AttributesFormatString=-----------------------------\n%<Gain>
  PS-Simulink Converter : nesl_utility/PS-Simulink Converter  PhysicalDomain=network_engine_domain  SubClassName=ps_output  LeftPortType=input  RightPortType=output  PseudoPeriodic=off  Frequencies=[]  Unit=A  AffineConversion=off
  PS-Simulink Converter1 : nesl_utility/PS-Simulink Converter  PhysicalDomain=network_engine_domain  SubClassName=ps_output  LeftPortType=input  RightPortType=output  PseudoPeriodic=off  Frequencies=[]  Unit=rad  AffineConversion=off
  PS-Simulink Converter2 : nesl_utility/PS-Simulink Converter  PhysicalDomain=network_engine_domain  SubClassName=ps_output  LeftPortType=input  RightPortType=output  PseudoPeriodic=off  Frequencies=[]  Unit=N*m  AffineConversion=off
  PS-Simulink Converter3 : nesl_utility/PS-Simulink Converter  PhysicalDomain=network_engine_domain  SubClassName=ps_output  LeftPortType=input  RightPortType=output  PseudoPeriodic=off  Frequencies=[]  Unit=rad/s  AffineConversion=off
  Park Transform : eeTransforms/Park Transform  AxisAlignment=D-axis  PowerInvariant=off
  Terminator : Terminator
  C : PMIOPort  Side=Left
  T : PMIOPort  Port=2  Side=Left
  A : PMIOPort  Port=3  Side=Left
  W : PMIOPort  Port=4  Side=Left
  M : Outport  OutDataTypeStr=Bus: motorMeasurements  VectorParamsAs1DForOutWhenUnconnected=off
  wires:
  Demux/2 -> Bus_Creator2/2  "phaseCurrentB"
  Demux/3 -> Bus_Creator2/3  "phaseCurrentC"
  Demux/1 -> Bus_Creator2/1  "phaseCurrentA"
  PS-Simulink Converter/1 -> Park Transform/1, Demux/1
  Bus_Creator2/1 -> M/1
  PS-Simulink Converter2/1 -> Bus_Creator2/6  "electromagneticTorque"
  PS-Simulink Converter3/1 -> Bus_Creator2/9, Gain2/1  "rotorVelocity"
  PS-Simulink Converter1/1 -> Bus_Creator2/7, Gain1/1  "rotorPosition"
  Gain1/1 -> Park Transform/2, Bus_Creator2/8  "electricalPosition"
  Gain2/1 -> Bus_Creator2/10  "electricalVelocity"
  Demux1/1 -> Bus_Creator2/4  "directCurrent"
  Demux1/2 -> Bus_Creator2/5  "quadratureCurrent"
  Park Transform/1 -> Demux1/1
  Demux1/3 -> Terminator/1
  connections:
  PS-Simulink Converter/LConn1 -- C/RConn1
  PS-Simulink Converter1/LConn1 -- A/RConn1
  PS-Simulink Converter2/LConn1 -- T/RConn1
  PS-Simulink Converter3/LConn1 -- W/RConn1

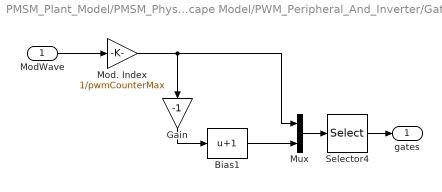
== system PMSM_Plant_Model/PMSM_Physical_Model/PMSM Simscape Model/PWM_Peripheral_And_Inverter/Gate driver ==
  ModWave : Inport
  Bias1 : Bias  Bias=1
  Gain : Gain  Gain=-1
  Mod. Index : Gain  Gain=1/pwmCounterMax  OutDataTypeStr=Inherit: Inherit via back propagation
  Mux : Mux  Inputs=2
  Selector4 : Selector  InputPortWidth=6  IndexOptions=Index vector (dialog)  Indices=[1 4 2 5 3 6]  OutputSizes=1
  gates : Outport
  wires:
  Selector4/1 -> gates/1
  Mux/1 -> Selector4/1
  ModWave/1 -> Mod. Index/1
  Gain/1 -> Bias1/1
  Bias1/1 -> Mux/2
  Mod. Index/1 -> Gain/1, Mux/1
